simulink model "test01"  (Simulink 7.4)
settings: Solver=ode45  StartTime=0.0  StopTime=10.0  RelTol=1e-3
libraries: NAV420Lib x1
settings Model: Creator=djulzz  LastModifiedBy=autopilot

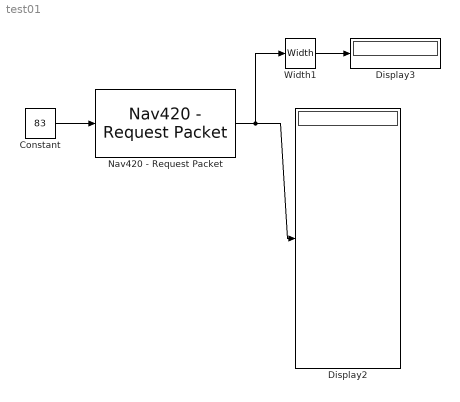
== system test01 ==
  Constant : Constant  Value=83  OutDataTypeMode=int8  OutDataType=fixdt(1, 16)  OutScaling=2^0  OutDataTypeStr=int8
  Display2 : Display
      settings: Format=hex (Stored Integer)
  Display3 : Display
  Nav420 - Request Packet : NAV420Lib/Nav420 - Request Packet  SystemSampleTime=-1
  Width1 : Width
  wires:
  Nav420 - Request Packet/1 -> Display2/1, Width1/1
  Width1/1 -> Display3/1
  Constant/1 -> Nav420 - Request Packet/1
